simulink model "pid_motor_modelo"  (R2015b)
settings: Solver=VariableStepAuto  StartTime=0.0  StopTime=6  RelTol=1e-3
settings Model: Creator=nico  LastModifiedBy=nico

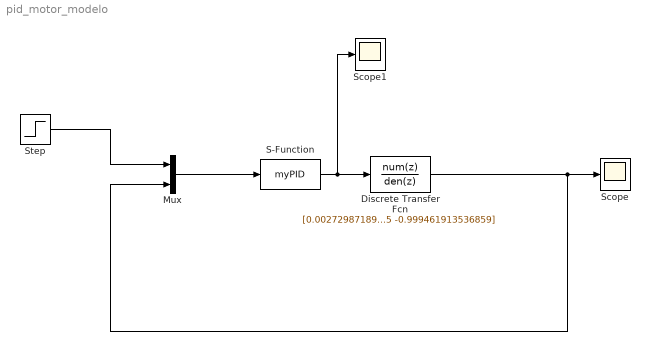
== system pid_motor_modelo ==
  Discrete Transfer Fcn : DiscreteTransferFcn  Numerator=[0.002729871894989]  Denominator=[1 -8.605285413471888e-05 -0.999461913536859]
  Mux : Mux  Inputs=2
  S-Function : S-Function  FunctionName=myPID  Parameters=1.2 0.01 4 10 .0001 0 24  SFunctionDeploymentMode=off  EnableBusSupport=off
  Scope : Scope
  Scope1 : Scope
  Step : Step  Time=0.2  After=75  SampleTime=0
  wires:
  Mux/1 -> S-Function/1
  Step/1 -> Mux/1
  S-Function/1 -> Discrete Transfer Fcn/1, Scope1/1
  Discrete Transfer Fcn/1 -> Mux/2, Scope/1
